simulink model "mybldc_mdl2"  (Simulink 10.0)
settings: Solver=ode113  StartTime=0.0  StopTime=.13  RelTol=1e-3  EnableMultiTasking=on
settings Model: Creator=bhisma  LastModifiedBy=bhisma
settings DataIOCC: SignalLoggingSaveFormat=ModelDataLogs  SignalLoggingName=sigsOut
settings OptimizationCC: BlockReduction=off  BooleanDataType=off  LifeSpan=auto
settings DebuggingCC: SaveWithParameterizedLinksMsg=none  SignalResolutionControl=TryResolveAllWithWarning  MultiTaskDSMMsg=warning  MultiTaskCondExecSysMsg=none  SFUnexpectedBacktrackingDiag=error  SFNoUnconditionalDefaultTransitionDiag=error  SFExecutionAtInitializationDiag=warning  ArithmeticOperatorsInVariantConditions=error
settings HardwareCC: TargetUnknown=on
settings SFSimCC: SimUseLocalCustomCode=on  SimParseCustomCode=off  CustomCodeUndefinedFunction=FilterOut
settings RTWCC: RTWUseLocalCustomCode=on
settings CodeAppCC: StateflowObjectComments=off
settings GRTTargetCC: TargetLangStandard=C99 (ISO)

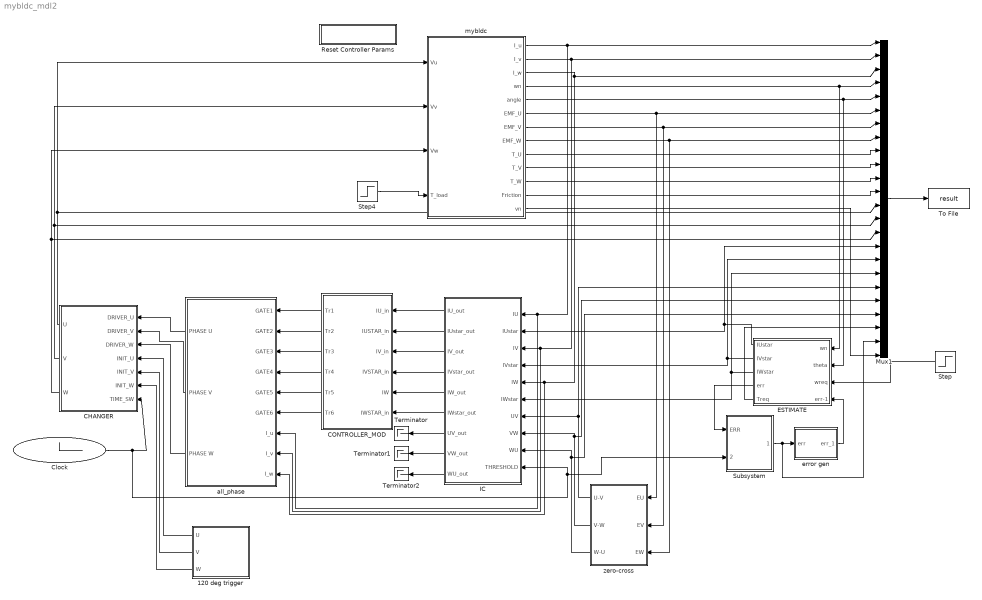
== system mybldc_mdl2 ==
  120 deg trigger : Subsystem  mask{T=1/50, V=160}
      mask prompts: T "Time period"; V "Excitation Voltage"
      mask help: This block is used to ramp up the motor.
  CHANGER : Subsystem  mask{T=400e-6}
      mask prompts: T "Threshold time"
      mask help:
      | This block is used to switch the bldc operation from an open loop to an initial one.
      | Fill in the amount of time bldc is to be run under open loop condition in the field
      | 'Threshold time'
      mask Help:
      | The controller by itself cannot start the motor. This is because the controller operation
      | is heavily dependent upon the Back EMF (BEMF) voltages. Initially, the rotor is at
      | standstill, and the back emf voltages have not built up. Thus, the controller does not
      | have any synchronizing information.
      | 
      | Therefore, for some inital time called the 'threshold time' , the motor is 'blindly' ramped
      | up. This is done by the '120 deg trigger' block which forces the 6 step commutation
      | sequence on the motor.
      | 
      | After the 'threshold time' sufficient back emf voltages have built up and then the 'CHANGER'
      | block just puts the BLDC motor into the closed loop operation.
      | 
      | For more information refer to the accompanying manual.
  CONTROLLER_MOD : Subsystem
  Clock : Clock
  ESTIMATE : Subsystem  mask{N=100, BM=49/60, J=0.0002, DF=0.002, Rr=0.02, Rl=0.03, delta=0, KP=50000, KI=500000, KD=5, basecurr=34}
      mask prompts: N "Number of turns per phase"; BM "Maximum value of magnetic field intensity"; J "moment of inertia"; DF "viscous friction"; Rr "Rotor radius"; Rl "Rotor length"; delta "phase difference between current and torque"; KP "Proportionality constant"; KI "Integral constant"; KD "differential constant"; basecurr "rated base current"
      mask help:
      | This block calculates the required calue of current in all the three phases depending upon the speed requirement
      |
      | For good results, phase difference should be kept at 0
      mask Help:
      | The estimation block calculates the currents that should be flowing in the individual
      | phases as per the speed command and/or the load torque requirements. For this a
      | PID controller is used. A series of transformations is applied in the m file s fuction
      | 'calc_core.m' and then commands are calculated. A modified version of the Park's
      | Transform is used. The signals are then fed to the controller block to decide the
      | appropriate switching strategy. For more details, refer to the accompanykng manual
  IC : Subsystem  mask{T=400e-6}
      mask prompts: T "Threshold"
      mask help:
      | The block is just used to hold the FSM in CONTROLLER_MOD block to its
      | inital states. The value in the field 'Threshold' determines how long the block
      | will keep the CONTROLLER_MOD block locked to its initial position.
      mask Help:
      | Intially, when the motor is being ramped to build up the required Back emf voltages,
      | it is important that the FSMs in the CONTROLLER_MOD block do not leave their
      | initial states. Therefore, this block is used to keep the FSMs in the CONTROLLER_MOD
      | block locked into their initial states. The time for which this control is exercised is
      | determined by the time value entered in 'Threshold' field.
      | Also, it is important that the same threshold value be entered in 'CHANGER', 'SUNSYSTEM'
      | and the 'IC' blocks.
  Mux1 : Mux  Inputs=24
  Reset Controller Params : Subsystem
      settings: OpenFcn=mybldc2([],[],[],'reset',find_system(get_param(gcs,'Handle'),'LookUnderMasks','all','Tag','PPC'));
      mask Display: disp('Reset Controller')
  Step : Step  Time=0.01  After=75  SampleTime=0
  Step4 : Step  Time=0.05  After=0  SampleTime=0
  Subsystem : Subsystem  mask{T=400e-6}
      mask prompts: T "Threshold"
  Terminator : Terminator
  Terminator1 : Terminator
  Terminator2 : Terminator
  To File : ToFile  Filename=result  MatrixName=res
  all_phase : Subsystem  mask{BV=160}
      mask prompts: BV "Battery voltage for excitation"
      mask help: This is an inverter. Double click the block to enter the battery voltage
      mask Help:
      | The voltage source that is used is bipolar. That is if a value say 100 is entered then a split supply
      | of +100 and -100 volts is assumed with respect to ground (zero volts)
  error gen : Subsystem
  mybldc : Subsystem
  zero-cross : Subsystem
      mask help: The block detects the zero crossing of the inputs. For accurate results use the rising edge only.
      mask Help:
      | The block determines t he zero crossing of (U-V) BEMF; (V-W) BEMF; (W-U) BEMFs.
      | It may be noted that SIMULINK determines its own step size (if allowed to ) and therefore
      | explicit zeros may not be reported in the solution. For example, the solution at consecutive
      | time steps may be -0.9 -0.95 +0.01...Hence there is an 'implied' zero crossing. The
      | Simulator was initially written in R12 where zero crossing detection block was not available
      | However, before replacing this block with the equivalent SIMULINK block, a functional
      | verification should be carried out.
  wires:
  Step4/1 -> mybldc/4(T_load)
  error gen/1(err_1) -> ESTIMATE/4(err-1)
  120 deg trigger/1(U) -> CHANGER/4(INIT_U)
  120 deg trigger/2(V) -> CHANGER/5(INIT_V)
  120 deg trigger/3(W) -> CHANGER/6(INIT_W)
  Clock/1 -> CHANGER/7(TIME_SW), IC/10(THRESHOLD), Subsystem/2(THRESHOLD)
  CHANGER/1(U) -> mybldc/1(Vu), Mux1/13
  CHANGER/2(V) -> mybldc/2(Vv), Mux1/14
  CHANGER/3(W) -> mybldc/3(Vw), Mux1/15
  ESTIMATE/1(IUstar) -> IC/2(IUstar), Mux1/16
  ESTIMATE/2(IVstar) -> IC/4(IVstar), Mux1/17
  ESTIMATE/3(IWstar) -> IC/6(IWstar), Mux1/18
  zero-cross/1(U-V) -> IC/7(UV), Mux1/19
  zero-cross/2(V-W) -> IC/8(VW), Mux1/20
  zero-cross/3(W-U) -> IC/9(WU), Mux1/21
  mybldc/1(I_u) -> Mux1/1, IC/1(IU), all_phase/7(I_u)
  mybldc/2(I_v) -> Mux1/2, IC/3(IV), all_phase/8(I_v)
  mybldc/3(I_w) -> Mux1/3, IC/5(IW), all_phase/9(I_w)
  mybldc/4(wn) -> Mux1/4, ESTIMATE/1(wn)
  mybldc/5(angle) -> Mux1/5, ESTIMATE/2(theta)
  mybldc/6(EMF_U) -> Mux1/6, zero-cross/1(EU)
  mybldc/7(EMF_V) -> Mux1/7, zero-cross/2(EV)
  mybldc/8(EMF_W) -> Mux1/8, zero-cross/3(EW)
  mybldc/9(T_U) -> Mux1/9
  mybldc/10(T_V) -> Mux1/10
  mybldc/11(T_W) -> Mux1/11
  mybldc/12(Friction) -> Mux1/12
  Mux1/1 -> To File/1
  ESTIMATE/5(Treq) -> Mux1/22
  Subsystem/1(ERR_out) -> error gen/1(err), Mux1/23
  ESTIMATE/4(err) -> Subsystem/1(ERR)
  all_phase/1(PHASE U) -> CHANGER/1(DRIVER_U)
  all_phase/2(PHASE V) -> CHANGER/2(DRIVER_V)
  all_phase/3(PHASE W) -> CHANGER/3(DRIVER_W)
  mybldc/13(vn) -> Mux1/24
  IC/1(IU_out) -> CONTROLLER_MOD/1(IU_in)
  IC/4(IVstar_out) -> CONTROLLER_MOD/4(IVSTAR_in)
  IC/5(IW_out) -> CONTROLLER_MOD/5(IW)
  IC/6(IWstar_out) -> CONTROLLER_MOD/6(IWSTAR_in)
  IC/7(UV_out) -> Terminator/1
  IC/8(VW_out) -> Terminator1/1
  IC/9(WU_out) -> Terminator2/1
  IC/3(IV_out) -> CONTROLLER_MOD/3(IV_in)
  IC/2(IUstar_out) -> CONTROLLER_MOD/2(IUSTAR_in)
  CONTROLLER_MOD/6(Tr6) -> all_phase/6(GATE6)
  CONTROLLER_MOD/5(Tr5) -> all_phase/5(GATE5)
  CONTROLLER_MOD/4(Tr4) -> all_phase/4(GATE4)
  CONTROLLER_MOD/3(Tr3) -> all_phase/3(GATE3)
  CONTROLLER_MOD/2(Tr2) -> all_phase/2(GATE2)
  CONTROLLER_MOD/1(Tr1) -> all_phase/1(GATE1)
  Step/1 -> ESTIMATE/3(wreq)

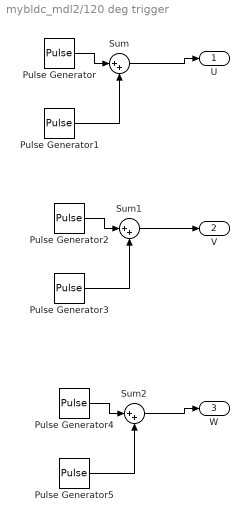
== system mybldc_mdl2/120 deg trigger ==
  Pulse Generator : DiscretePulseGenerator  PulseType=Time based  Amplitude=V  Period=T  PulseWidth=200/3  PhaseDelay=T/3
  Pulse Generator1 : DiscretePulseGenerator  PulseType=Time based  Amplitude=-2*V  Period=2*T  PulseWidth=100/3  PhaseDelay=-2*T/3
  Pulse Generator2 : DiscretePulseGenerator  PulseType=Time based  Amplitude=V  Period=T  PulseWidth=200/3
  Pulse Generator3 : DiscretePulseGenerator  PulseType=Time based  Amplitude=-2*V  Period=2*T  PulseWidth=100/3
  Pulse Generator4 : DiscretePulseGenerator  PulseType=Time based  Amplitude=V  Period=T  PulseWidth=200/3  PhaseDelay=-T/3
  Pulse Generator5 : DiscretePulseGenerator  PulseType=Time based  Amplitude=-2*V  Period=2*T  PulseWidth=100/3  PhaseDelay=2*T/3
  Sum : Sum  Inputs=|++  SaturateOnIntegerOverflow=on  InputSameDT=on  OutDataTypeStr=Inherit: Same as first input
  Sum1 : Sum  Inputs=|++  SaturateOnIntegerOverflow=on  InputSameDT=on  OutDataTypeStr=Inherit: Same as first input
  Sum2 : Sum  Inputs=|++  SaturateOnIntegerOverflow=on  InputSameDT=on  OutDataTypeStr=Inherit: Same as first input
  U : Outport
  V : Outport  Port=2
  W : Outport  Port=3
  wires:
  Pulse Generator/1 -> Sum/1
  Pulse Generator1/1 -> Sum/2
  Pulse Generator2/1 -> Sum1/1
  Pulse Generator3/1 -> Sum1/2
  Pulse Generator4/1 -> Sum2/1
  Pulse Generator5/1 -> Sum2/2
  Sum/1 -> U/1
  Sum1/1 -> V/1
  Sum2/1 -> W/1

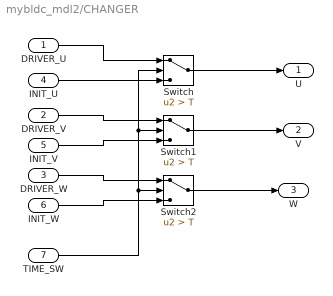
== system mybldc_mdl2/CHANGER ==
  DRIVER_U : Inport
  DRIVER_V : Inport  Port=2
  DRIVER_W : Inport  Port=3
  INIT_U : Inport  Port=4
  INIT_V : Inport  Port=5
  INIT_W : Inport  Port=6
  TIME_SW : Inport  Port=7
  Switch : Switch  Criteria=u2 > Threshold  Threshold=T  SaturateOnIntegerOverflow=on
  Switch1 : Switch  Criteria=u2 > Threshold  Threshold=T  SaturateOnIntegerOverflow=on
  Switch2 : Switch  Criteria=u2 > Threshold  Threshold=T  SaturateOnIntegerOverflow=on
  U : Outport
  V : Outport  Port=2
  W : Outport  Port=3
  wires:
  DRIVER_U/1 -> Switch/1
  DRIVER_V/1 -> Switch1/1
  DRIVER_W/1 -> Switch2/1
  INIT_U/1 -> Switch/3
  INIT_V/1 -> Switch1/3
  INIT_W/1 -> Switch2/3
  TIME_SW/1 -> Switch/2, Switch1/2, Switch2/2
  Switch2/1 -> W/1
  Switch1/1 -> V/1
  Switch/1 -> U/1

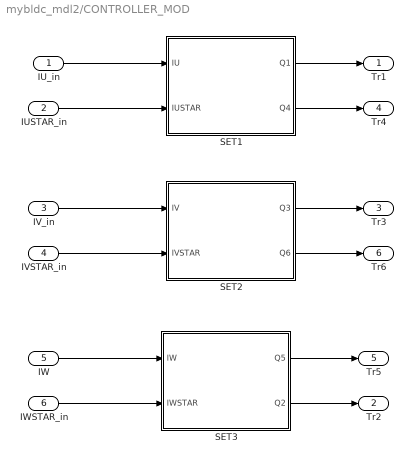
== system mybldc_mdl2/CONTROLLER_MOD ==
  IU_in : Inport
  IUSTAR_in : Inport  Port=2
  IV_in : Inport  Port=3
  IVSTAR_in : Inport  Port=4
  IW : Inport  Port=5
  IWSTAR_in : Inport  Port=6
  SET1 : Stateflow chart  TreatAsAtomicUnit=on
  SET2 : Stateflow chart  TreatAsAtomicUnit=on
  SET3 : Stateflow chart  TreatAsAtomicUnit=on
  Tr1 : Outport
  Tr2 : Outport  Port=2
  Tr3 : Outport  Port=3
  Tr4 : Outport  Port=4
  Tr5 : Outport  Port=5
  Tr6 : Outport  Port=6
  wires:
  IU_in/1 -> SET1/1(IU)
  IUSTAR_in/1 -> SET1/2(IUSTAR)
  IV_in/1 -> SET2/1(IV)
  IVSTAR_in/1 -> SET2/2(IVSTAR)
  IW/1 -> SET3/1(IW)
  IWSTAR_in/1 -> SET3/2(IWSTAR)
  SET1/1(Q1) -> Tr1/1
  SET3/2(Q2) -> Tr2/1
  SET2/1(Q3) -> Tr3/1
  SET1/2(Q4) -> Tr4/1
  SET3/1(Q5) -> Tr5/1
  SET2/2(Q6) -> Tr6/1

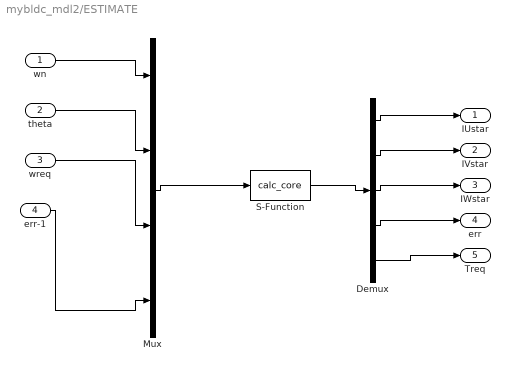
== system mybldc_mdl2/ESTIMATE ==
  wn : Inport
  theta : Inport  Port=2
  wreq : Inport  Port=3
  err-1 : Inport  Port=4
  Demux : Demux  Outputs=5
  Mux : Mux
  S-Function : S-Function  FunctionName=calc_core  Parameters=J,DF,N,BM,Rr,Rl,delta,KP,KI,KD,basecurr  SFunctionDeploymentMode=off  EnableBusSupport=off
  IUstar : Outport
  IVstar : Outport  Port=2
  IWstar : Outport  Port=3
  err : Outport  Port=4
  Treq : Outport  Port=5
  wires:
  S-Function/1 -> Demux/1
  Mux/1 -> S-Function/1
  err-1/1 -> Mux/4
  wreq/1 -> Mux/3
  theta/1 -> Mux/2
  wn/1 -> Mux/1
  Demux/4 -> err/1
  Demux/3 -> IWstar/1
  Demux/2 -> IVstar/1
  Demux/1 -> IUstar/1
  Demux/5 -> Treq/1

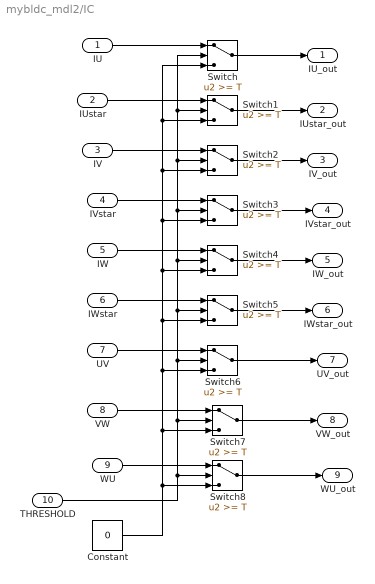
== system mybldc_mdl2/IC ==
  IU : Inport
  IUstar : Inport  Port=2
  IV : Inport  Port=3
  IVstar : Inport  Port=4
  IW : Inport  Port=5
  IWstar : Inport  Port=6
  UV : Inport  Port=7
  VW : Inport  Port=8
  WU : Inport  Port=9
  THRESHOLD : Inport  Port=10
  Constant : Constant  Value=0
  Switch{,1..8} (9 alike) : Switch  Threshold=T  SaturateOnIntegerOverflow=on
  IU_out : Outport
  IUstar_out : Outport  Port=2
  IV_out : Outport  Port=3
  IVstar_out : Outport  Port=4
  IW_out : Outport  Port=5
  IWstar_out : Outport  Port=6
  UV_out : Outport  Port=7
  VW_out : Outport  Port=8
  WU_out : Outport  Port=9
  wires:
  IU/1 -> Switch/1
  IUstar/1 -> Switch1/1
  IV/1 -> Switch2/1
  IVstar/1 -> Switch3/1
  IW/1 -> Switch4/1
  IWstar/1 -> Switch5/1
  UV/1 -> Switch6/1
  VW/1 -> Switch7/1
  WU/1 -> Switch8/1
  Constant/1 -> Switch8/3, Switch7/3, Switch6/3, Switch5/3, Switch4/3, Switch3/3, Switch2/3, Switch1/3, Switch/3
  Switch/1 -> IU_out/1
  Switch1/1 -> IUstar_out/1
  Switch2/1 -> IV_out/1
  Switch3/1 -> IVstar_out/1
  Switch4/1 -> IW_out/1
  Switch5/1 -> IWstar_out/1
  Switch6/1 -> UV_out/1
  Switch7/1 -> VW_out/1
  Switch8/1 -> WU_out/1
  THRESHOLD/1 -> Switch/2, Switch1/2, Switch2/2, Switch3/2, Switch4/2, Switch5/2, Switch6/2, Switch7/2, Switch8/2

== system mybldc_mdl2/Reset Controller Params ==

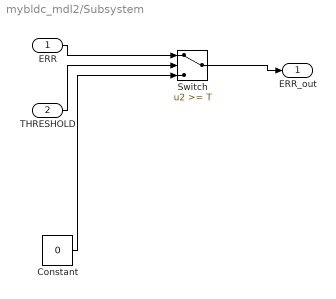
== system mybldc_mdl2/Subsystem ==
  ERR : Inport
  THRESHOLD : Inport  Port=2
  Constant : Constant  Value=0
  Switch : Switch  Threshold=T  SaturateOnIntegerOverflow=on
  ERR_out : Outport
  wires:
  ERR/1 -> Switch/1
  THRESHOLD/1 -> Switch/2
  Switch/1 -> ERR_out/1
  Constant/1 -> Switch/3

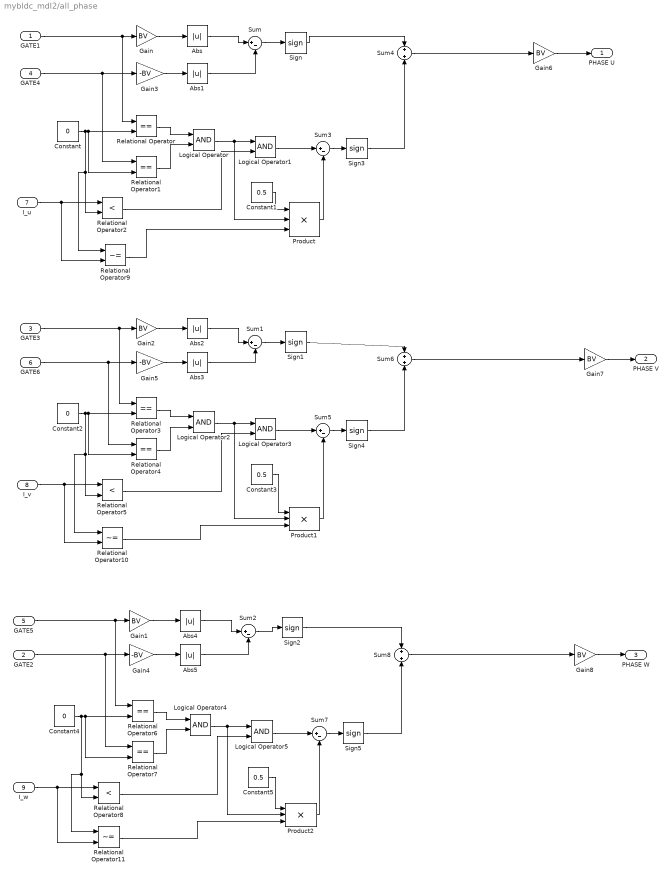
== system mybldc_mdl2/all_phase ==
  GATE1 : Inport
  GATE2 : Inport  Port=2
  GATE3 : Inport  Port=3
  GATE4 : Inport  Port=4
  GATE5 : Inport  Port=5
  GATE6 : Inport  Port=6
  I_u : Inport  Port=7
  I_v : Inport  Port=8
  I_w : Inport  Port=9
  Abs{,1..5} (6 alike) : Abs  SaturateOnIntegerOverflow=on
  Constant : Constant  Value=0
  Constant1 : Constant  Value=0.5
  Constant2 : Constant  Value=0
  Constant3 : Constant  Value=0.5
  Constant4 : Constant  Value=0
  Constant5 : Constant  Value=0.5
  Gain{,1..2,6..8} (6 alike) : Gain  Gain=BV  SaturateOnIntegerOverflow=on  OutDataTypeStr=Inherit: Same as input  ParamDataTypeStr=Inherit: Same as input
  Gain3 : Gain  Gain=-BV  SaturateOnIntegerOverflow=on  OutDataTypeStr=Inherit: Same as input  ParamDataTypeStr=Inherit: Same as input
  Gain4 : Gain  Gain=-BV  SaturateOnIntegerOverflow=on  OutDataTypeStr=Inherit: Same as input  ParamDataTypeStr=Inherit: Same as input
  Gain5 : Gain  Gain=-BV  SaturateOnIntegerOverflow=on  OutDataTypeStr=Inherit: Same as input  ParamDataTypeStr=Inherit: Same as input
  Logical Operator{,1..5} (6 alike) : Logic  AllPortsSameDT=off
  Product : Product  Inputs=3  SaturateOnIntegerOverflow=on  OutDataTypeStr=Inherit: Same as first input
  Product1 : Product  Inputs=3  SaturateOnIntegerOverflow=on  OutDataTypeStr=Inherit: Same as first input
  Product2 : Product  Inputs=3  SaturateOnIntegerOverflow=on  OutDataTypeStr=Inherit: Same as first input
  Relational Operator{,1,3..4,6..7} (6 alike) : RelationalOperator  Operator===  RndMeth=Nearest
  Relational Operator10 : RelationalOperator  Operator=~=  RndMeth=Nearest
  Relational Operator11 : RelationalOperator  Operator=~=  RndMeth=Nearest
  Relational Operator2 : RelationalOperator  Operator=<  RndMeth=Nearest
  Relational Operator5 : RelationalOperator  Operator=<  RndMeth=Nearest
  Relational Operator8 : RelationalOperator  Operator=<  RndMeth=Nearest
  Relational Operator9 : RelationalOperator  Operator=~=  RndMeth=Nearest
  Sign{,1..5} (6 alike) : Signum
  Sum{,1..3,5,7} (6 alike) : Sum  Inputs=|+-  SaturateOnIntegerOverflow=on  InputSameDT=on  OutDataTypeStr=Inherit: Same as first input
  Sum4 : Sum  SaturateOnIntegerOverflow=on  InputSameDT=on  OutDataTypeStr=Inherit: Same as first input
  Sum6 : Sum  SaturateOnIntegerOverflow=on  InputSameDT=on  OutDataTypeStr=Inherit: Same as first input
  Sum8 : Sum  SaturateOnIntegerOverflow=on  InputSameDT=on  OutDataTypeStr=Inherit: Same as first input
  PHASE U : Outport
  PHASE V : Outport  Port=2
  PHASE W : Outport  Port=3
  wires:
  GATE1/1 -> Gain/1, Relational Operator/1
  GATE5/1 -> Gain1/1, Relational Operator6/1
  GATE3/1 -> Gain2/1, Relational Operator3/1
  GATE4/1 -> Gain3/1, Relational Operator1/1
  GATE2/1 -> Gain4/1, Relational Operator7/1
  GATE6/1 -> Gain5/1, Relational Operator4/1
  Gain/1 -> Abs/1
  Gain3/1 -> Abs1/1
  Gain2/1 -> Abs2/1
  Gain5/1 -> Abs3/1
  Gain1/1 -> Abs4/1
  Gain4/1 -> Abs5/1
  Abs/1 -> Sum/1
  Abs1/1 -> Sum/2
  Abs2/1 -> Sum1/1
  Abs3/1 -> Sum1/2
  Abs4/1 -> Sum2/1
  Abs5/1 -> Sum2/2
  Sum/1 -> Sign/1
  Sum1/1 -> Sign1/1
  Sum2/1 -> Sign2/1
  Gain8/1 -> PHASE W/1
  Gain7/1 -> PHASE V/1
  Gain6/1 -> PHASE U/1
  Constant/1 -> Relational Operator/2, Relational Operator1/2, Relational Operator2/2, Relational Operator9/1
  Relational Operator/1 -> Logical Operator/1
  Relational Operator1/1 -> Logical Operator/2
  I_u/1 -> Relational Operator2/1, Relational Operator9/2
  Logical Operator/1 -> Logical Operator1/1, Product/2
  Relational Operator2/1 -> Logical Operator1/2
  Logical Operator1/1 -> Sum3/1
  Sum3/1 -> Sign3/1
  Sign/1 -> Sum4/1
  Sign3/1 -> Sum4/2
  Sum4/1 -> Gain6/1
  Constant2/1 -> Relational Operator4/2, Relational Operator3/2, Relational Operator5/2, Relational Operator10/1
  Relational Operator3/1 -> Logical Operator2/1
  Relational Operator4/1 -> Logical Operator2/2
  I_v/1 -> Relational Operator5/1, Relational Operator10/2
  Logical Operator2/1 -> Logical Operator3/1, Product1/2
  Relational Operator5/1 -> Logical Operator3/2
  Logical Operator3/1 -> Sum5/1
  Sum5/1 -> Sign4/1
  Sign1/1 -> Sum6/1
  Sign4/1 -> Sum6/2
  Sum6/1 -> Gain7/1
  Constant4/1 -> Relational Operator6/2, Relational Operator7/2, Relational Operator8/2, Relational Operator11/1
  Relational Operator6/1 -> Logical Operator4/1
  Relational Operator7/1 -> Logical Operator4/2
  I_w/1 -> Relational Operator8/1, Relational Operator11/2
  Logical Operator4/1 -> Logical Operator5/1, Product2/2
  Relational Operator8/1 -> Logical Operator5/2
  Logical Operator5/1 -> Sum7/1
  Sum7/1 -> Sign5/1
  Sign5/1 -> Sum8/2
  Sign2/1 -> Sum8/1
  Sum8/1 -> Gain8/1
  Constant1/1 -> Product/1
  Product/1 -> Sum3/2
  Constant3/1 -> Product1/1
  Product1/1 -> Sum5/2
  Constant5/1 -> Product2/1
  Product2/1 -> Sum7/2
  Relational Operator9/1 -> Product/3
  Relational Operator10/1 -> Product1/3
  Relational Operator11/1 -> Product2/3

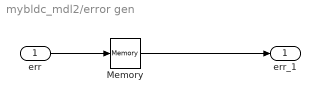
== system mybldc_mdl2/error gen ==
  err : Inport
  Memory : Memory  InheritSampleTime=on
  err_1 : Outport
  wires:
  Memory/1 -> err_1/1
  err/1 -> Memory/1

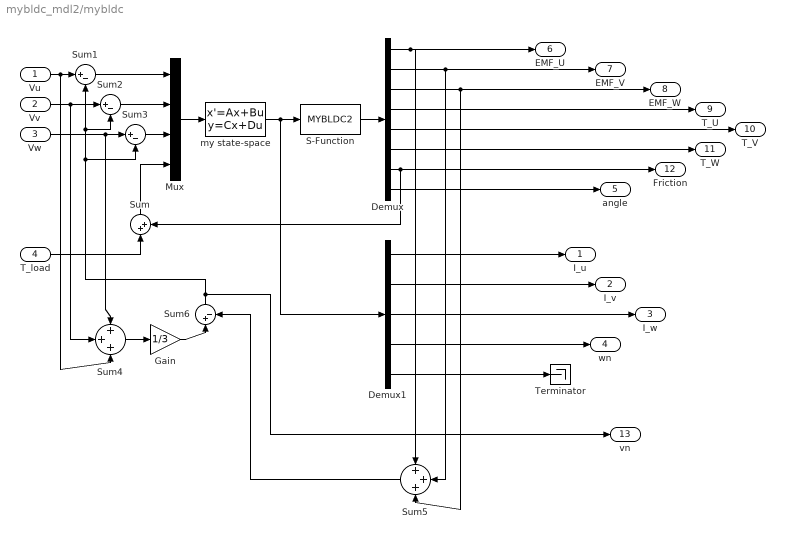
== system mybldc_mdl2/mybldc ==
  Vu : Inport
  Vv : Inport  Port=2
  Vw : Inport  Port=3
  T_load : Inport  Port=4
  Demux : Demux  Outputs=8
  Demux1 : Demux  Outputs=5
  Gain : Gain  Gain=1/3  SaturateOnIntegerOverflow=on  OutDataTypeStr=Inherit: Same as input  ParamDataTypeStr=Inherit: Same as input
  Mux : Mux
  S-Function : S-Function  FunctionName=MYBLDC2  Parameters=N,R,L,M,BM,Rl,Rr,DF,J,P,F0,Fs  SFunctionDeploymentMode=off  EnableBusSupport=off  mask{N=100, R=0.7, L=2.72e-3, M=-1.5e-3, BM=49/60, Rl=0.03, Rr=0.02, DF=0.002, J=0.0002, P=4, Fs=0.2*0.089, F0=0.089}
      mask prompts: N "Number of turns per phase"; R "Resistance per phase"; L "self inductance per phase"; M "mutual inductace per phase"; BM "Maximum value of flux density"; Rl "Rotor length"; Rr "rotor radius"; DF "value of viscous friction"; J "moment of inertia"; P "Total number of poles"; Fs "starting value of coulomb friction"; F0 "Static friction"
      mask help: The blovk post- processes the state space block outputs
      mask Help:
      | Many other variables like the back emf , normalised angles (to 2*pi) and friction are
      | calculated here. The block is essentially an m file S function 'mybldc2.m' wherein
      | the flux distribution has been written as a look up table and the values are calculated
      | using that look up table. For math, refer to the manual.
  Sum : Sum  Inputs=|++  SaturateOnIntegerOverflow=on  InputSameDT=on  OutDataTypeStr=Inherit: Same as first input
  Sum{1..3,6} (4 alike) : Sum  Inputs=|+-  SaturateOnIntegerOverflow=on  InputSameDT=on  OutDataTypeStr=Inherit: Same as first input
  Sum4 : Sum  Inputs=+++  SaturateOnIntegerOverflow=on  InputSameDT=on  OutDataTypeStr=Inherit: Same as first input
  Sum5 : Sum  Inputs=+++  SaturateOnIntegerOverflow=on  InputSameDT=on  OutDataTypeStr=Inherit: Same as first input
  Terminator : Terminator
  my state-space : StateSpace  A="[ -1.658768e+002  0 0 1.604892e-016 0; 0  -1.658768e+002 0 1.161137e+001 0; 0  0 -1.658768e+002 -1.161137e+001 0; -3.386321e-015  -245 245 -10 0; 0  0 0 2 0]"  B=[236.96 0 0 0; 0 236.96 0 0; 0 0 236.96 0; 0 0 0 -5000; 0 0 0 0]  C=[1 0 0 0 0;0 1 0 0 0;0 0 1 0 0; 0 0 0 1 0;0 0 0 0 1]  D=[0 0 0 0 ; 0 0 0 0; 0 0 0 0; 0 0 0 0; 0 0 0 0]  InitialCondition=[0 0 0 0 0]
  I_u : Outport
  I_v : Outport  Port=2
  I_w : Outport  Port=3
  wn : Outport  Port=4
  angle : Outport  Port=5
  EMF_U : Outport  Port=6
  EMF_V : Outport  Port=7
  EMF_W : Outport  Port=8
  T_U : Outport  Port=9
  T_V : Outport  Port=10
  T_W : Outport  Port=11
  Friction : Outport  Port=12
  vn : Outport  Port=13
  wires:
  Mux/1 -> my state-space/1
  my state-space/1 -> S-Function/1, Demux1/1
  S-Function/1 -> Demux/1
  Demux1/1 -> I_u/1
  Demux/1 -> EMF_U/1, Sum5/1
  Demux/2 -> EMF_V/1, Sum5/2
  Demux/3 -> EMF_W/1, Sum5/3
  Demux/4 -> T_U/1
  Demux/5 -> T_V/1
  Demux/6 -> T_W/1
  Demux/7 -> Friction/1, Sum/2
  Demux/8 -> angle/1
  Demux1/2 -> I_v/1
  Demux1/3 -> I_w/1
  Demux1/4 -> wn/1
  Demux1/5 -> Terminator/1
  Sum/1 -> Mux/4
  T_load/1 -> Sum/1
  Vu/1 -> Sum1/1, Sum4/3
  Sum1/1 -> Mux/1
  Vv/1 -> Sum2/1, Sum4/2
  Sum2/1 -> Mux/2
  Vw/1 -> Sum3/1, Sum4/1
  Sum3/1 -> Mux/3
  Sum4/1 -> Gain/1
  Gain/1 -> Sum6/1
  Sum5/1 -> Sum6/2
  Sum6/1 -> Sum1/2, Sum2/2, Sum3/2, vn/1

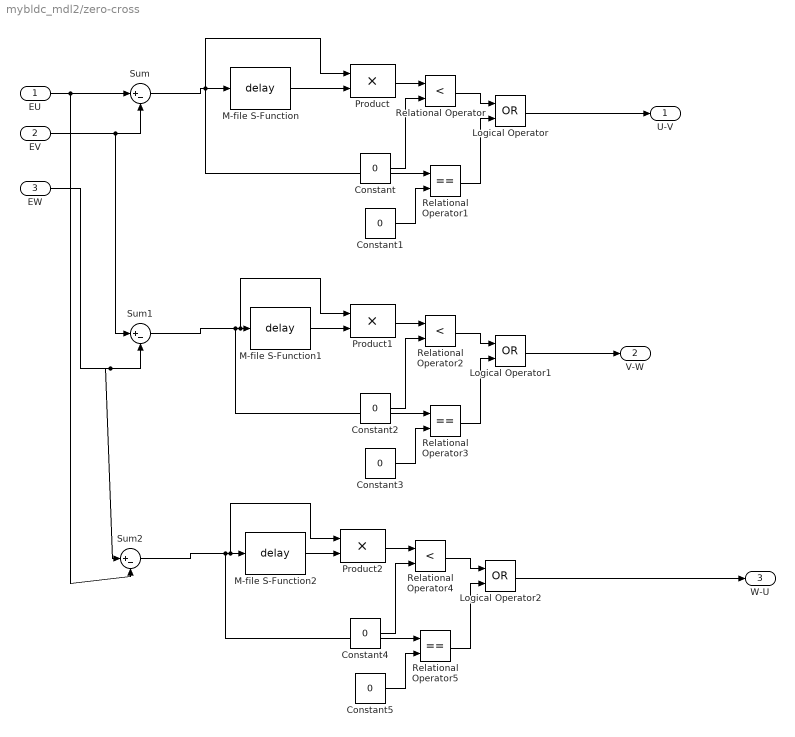
== system mybldc_mdl2/zero-cross ==
  EU : Inport
  EV : Inport  Port=2
  EW : Inport  Port=3
  Constant{,1..5} (6 alike) : Constant  Value=0
  Logical Operator : Logic  Operator=OR
  Logical Operator1 : Logic  Operator=OR
  Logical Operator2 : Logic  Operator=OR
  M-file S-Function : S-Function  FunctionName=delay  SFunctionDeploymentMode=off  EnableBusSupport=off  mask(S-function: sfun_dsc2){}
      mask help: This is a M-file S-function which demonstrates how toimplement an unit delay.
      mask Display: disp('Unit delay')
  M-file S-Function1 : S-Function  FunctionName=delay  SFunctionDeploymentMode=off  EnableBusSupport=off  mask(S-function: sfun_dsc2){}
      mask help: This is a M-file S-function which demonstrates how toimplement an unit delay.
      mask Display: disp('Unit delay')
  M-file S-Function2 : S-Function  FunctionName=delay  SFunctionDeploymentMode=off  EnableBusSupport=off  mask(S-function: sfun_dsc2){}
      mask help: This is a M-file S-function which demonstrates how toimplement an unit delay.
      mask Display: disp('Unit delay')
  Product : Product  SaturateOnIntegerOverflow=on  InputSameDT=on  OutDataTypeStr=Inherit: Same as first input
  Product1 : Product  SaturateOnIntegerOverflow=on  InputSameDT=on  OutDataTypeStr=Inherit: Same as first input
  Product2 : Product  SaturateOnIntegerOverflow=on  InputSameDT=on  OutDataTypeStr=Inherit: Same as first input
  Relational Operator : RelationalOperator  Operator=<  RndMeth=Nearest  InputSameDT=on
  Relational Operator1 : RelationalOperator  Operator===  RndMeth=Nearest  InputSameDT=on
  Relational Operator2 : RelationalOperator  Operator=<  RndMeth=Nearest  InputSameDT=on
  Relational Operator3 : RelationalOperator  Operator===  RndMeth=Nearest  InputSameDT=on
  Relational Operator4 : RelationalOperator  Operator=<  RndMeth=Nearest  InputSameDT=on
  Relational Operator5 : RelationalOperator  Operator===  RndMeth=Nearest  InputSameDT=on
  Sum : Sum  Inputs=|+-  SaturateOnIntegerOverflow=on  InputSameDT=on  OutDataTypeStr=Inherit: Same as first input
  Sum1 : Sum  Inputs=|+-  SaturateOnIntegerOverflow=on  InputSameDT=on  OutDataTypeStr=Inherit: Same as first input
  Sum2 : Sum  Inputs=|+-  SaturateOnIntegerOverflow=on  InputSameDT=on  OutDataTypeStr=Inherit: Same as first input
  U-V : Outport
  V-W : Outport  Port=2
  W-U : Outport  Port=3
  wires:
  Sum/1 -> Relational Operator1/1, Product/1, M-file S-Function/1
  M-file S-Function/1 -> Product/2
  Product/1 -> Relational Operator/1
  Constant/1 -> Relational Operator/2
  Constant1/1 -> Relational Operator1/2
  Relational Operator/1 -> Logical Operator/1
  Relational Operator1/1 -> Logical Operator/2
  Logical Operator/1 -> U-V/1
  EU/1 -> Sum/1, Sum2/2
  EV/1 -> Sum/2, Sum1/1
  Sum1/1 -> Relational Operator3/1, Product1/1, M-file S-Function1/1
  M-file S-Function1/1 -> Product1/2
  Product1/1 -> Relational Operator2/1
  Constant2/1 -> Relational Operator2/2
  Constant3/1 -> Relational Operator3/2
  Relational Operator2/1 -> Logical Operator1/1
  Relational Operator3/1 -> Logical Operator1/2
  Logical Operator1/1 -> V-W/1
  EW/1 -> Sum1/2, Sum2/1
  Sum2/1 -> M-file S-Function2/1, Product2/1, Relational Operator5/1
  M-file S-Function2/1 -> Product2/2
  Product2/1 -> Relational Operator4/1
  Constant4/1 -> Relational Operator4/2
  Constant5/1 -> Relational Operator5/2
  Relational Operator4/1 -> Logical Operator2/1
  Relational Operator5/1 -> Logical Operator2/2
  Logical Operator2/1 -> W-U/1

== stateflow chart CONTROLLER_MOD/SET1 ==
  settings: updateMethod=CONTINUOUS  executeAtInitialization=1
  state A/
    state A1/
      during:Q1=1;Q4=0;
    state A2/
      during:Q4=1;Q1=0;
    A2 -> A1 : [IU<IUSTAR]
    (default) -> A1 : [1]
    A1 -> A2 : [IU>IUSTAR]
  (default) -> A : [1]
  data: IU input double; IUSTAR input double; Q1 output double; Q4 output double

== stateflow chart CONTROLLER_MOD/SET2 ==
  settings: updateMethod=CONTINUOUS  executeAtInitialization=1
  state B/
    state B1/
      during:Q3=1;Q6=0;
    state B2/
      during:Q3=0;Q6=1;
    B2 -> B1 : [IV<IVSTAR]
    (default) -> B1 : [1]
    B1 -> B2 : [IV>IVSTAR]
  (default) -> B : [1]
  data: IV input double; IVSTAR input double; Q3 output double; Q6 output double

== stateflow chart CONTROLLER_MOD/SET3 ==
  settings: updateMethod=CONTINUOUS  executeAtInitialization=1
  state C/
    state C1/
      during:Q5=1;Q2=0;
    state C2/
      during:Q5=0;Q2=1;
    C2 -> C1 : [IW<IWSTAR]
    (default) -> C1 : [1]
    C1 -> C2 : [IW>IWSTAR]
  (default) -> C : [1]
  data: IW input double; IWSTAR input double; Q5 output double; Q2 output double
